simulink model "pendulum_motion"  (R2021a)
settings: Solver=VariableStepAuto  StartTime=0.0  StopTime=10.0  MaxStep=1e-3  RelTol=1e-3
undefined symbols (not defined in the file): g, inti_dis, inti_velo, L
settings Model: Creator=AHMED  LastModifiedBy=AHMED

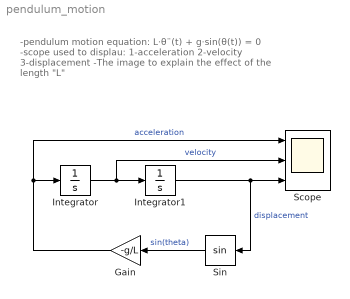
== system pendulum_motion ==
  note: -pendulum motion equation:
      | 	L⋅θ¨(t) + g⋅sin(θ(t)) = 0
      | -scope used to displau:
      | 	1-acceleration
      | 	2-velocity
      | 	3-displacement
      | -The image to explain the effect of the length "L"
  Gain : Gain  Gain=-g/L
  Integrator : Integrator  InitialCondition=inti_velo
  Integrator1 : Integrator  InitialCondition=inti_dis
  Scope : Scope  NumInputPorts=3
  Sin : Trigonometry
  wires:
  Integrator/1 -> Scope/2, Integrator1/1  "velocity"
  Integrator1/1 -> Scope/3, Sin/1  "displacement"
  Gain/1 -> Scope/1, Integrator/1  "acceleration"
  Sin/1 -> Gain/1  "sin(theta)"
